simulink model "E55_1030"  (R2019b)
settings: Solver=FixedStepDiscrete  StartTime=0.0  StopTime=10  FixedStep=0.0005  RelTol=1e-3  EnableMultiTasking=on
InitFcn:
  | ecucoder_canfd
  | load('DATA_Plimit.mat')
  | a=0.775;
  | b=0.775;
  | kf=-50000;
  | kr=-50000;
  | m=226+75;
  | Iz=100;
  | u=0.85;
  | g=9.8;
  | L=a+b;
  | xi=0.1;
  | r=0.226;
  | Lw=1.171;
  | Tm=21;
  | i=15.9;
  | Jw=0.504;
  | Pmax=20000;
  | mw=19.3;
  | mb=148.9+75;
  | hg=0.280;
model workspace (MAT data in the model file):
  Initial_Steer_Position = 0
values from neighbouring files (symbols this model uses):
  SOC = [2.5 5 7.5 10 20 30 40 50 60 70 80 90 ... (14 elements, 14x1)]    [DATA_Plimit.mat]
  SOC_Discharge = [2.04592350211 2.57821618825 3.10671863859 3.63118835861 4.15200192786 4.66837694959 5.18149950051 5.69046162564 6.19532286188 6.696400261 7.19347596839 7.68712157998 ... (473 elements, 1x473)]    [DATA_Plimit.mat]
  VOLTAGE = [459.1488 476.0844 485.9448 487.344 492.822 498.8016 503.382 509.1108 518.8128 531.2472 544.5132 558.4656 ... (14 elements, 14x1)]    [DATA_Plimit.mat]
undefined symbols (not defined in the file or in its folder): DiscIntNeverNeededParam, H, HALL10, HALL6, HALL7, HALL8, HALL9, HPWM1, HPWM3, I_AN05_5V, I_AN07_5V, I_AN08_5V, I_AN09_5V, I_AN10_5V, I_SW11_H, I_SW12_H, I_SW13_H, I_SW14_H, I_SW15_H, I_SW16_H, I_SW17_H, I_SW18_H, I_SW19_H, LS1A2, O_HS1A2, O_HS1A8
libraries: ec311lib x152, simulink x92, canmsglib x30, canfdmsglib x2
(part 1 of 6)
settings Model: PacingRate=0.100000  Creator=Bobbby  LastModifiedBy=Administrator
settings OptimizationCC: DefaultParameterBehavior=Inlined  InlineInvariantSignals=on  EnhancedBackFolding=on  ExpressionFolding=off  PassReuseOutputArgsAs=Individual arguments  RollThreshold=65  StateBitsets=on  DataBitsets=on  ZeroExternalMemoryAtStartup=off  ZeroInternalMemoryAtStartup=off  EfficientFloat2IntCast=on  OptimizeBlockOrder=speed  DifferentSizesBufferReuse=on  EfficientTunableParamExpr=on
settings DebuggingCC: InheritedTsInSrcMsg=none  ParameterTunabilityLossMsg=error  UnconnectedInputMsg=none  UnconnectedOutputMsg=none  UnconnectedLineMsg=none  SFMachineParentedDataDiag=error
settings HardwareCC: ProdBitPerPointer=32  ProdBitPerSizeT=32  ProdBitPerPtrDiffT=32  ProdLargestAtomicInteger=Long  ProdLargestAtomicFloat=Double  ProdWordSize=32  ProdHWDeviceType=ARM Compatible->ARM Cortex
settings SFSimCC: MATLABDynamicMemAlloc=off  CustomCodeUndefinedFunction=UseInterfaceOnly
settings RTWCC: Description=Target for EC311  SystemTargetFile=ec311.tlc  MakeCommand=make_rtw optimized_fixed_point=1  GenerateMakefile=off  TemplateMakefile=ec311_lcc.tmf  PostCodeGenCommand=ec311_pst_s2(buildInfo)  GenerateReport=on  IncludeHyperlinkInReport=on  LaunchReport=on
settings CodeAppCC: ForceParamTrailComments=on  IgnoreCustomStorageClasses=off  OperatorAnnotations=on  SimulinkDataObjDesc=on  SFDataObjDesc=on  InsertBlockDesc=on
settings STFCustomTargetCC: TargetLangStandard=C99 (ISO)  MultiwordLength=256  IncludeMdlTerminateFcn=off  CombineOutputUpdateFcns=on  SuppressErrorStatus=on  ERTCustomFileBanners=on  SupportNonFinite=off  SupportContinuousTime=off  SupportNonInlinedSFcns=off  RemoveResetFunc=on  MATLABClassNameForMDSCustomization=Simulink.SoftwareTarget.ERTCustomization  SystemTargetFile=ec311.tlc
settings ERTTargetCC: TargetLangStandard=C99 (ISO)  ParMdlRefBuildCompliant=off  CompOptLevelCompliant=off  ConcurrentExecutionCompliant=off  IncludeMdlTerminateFcn=off  SuppressErrorStatus=on  SupportNonFinite=off  ModelStepFunctionPrototypeControlCompliant=off  CPPClassGenCompliant=off  UseToolchainInfoCompliant=off  GenerateASAP2=on  InlinedParameterPlacement=NonHierarchical  ERTSrcFileBannerTemplate=ec311_code_template.cgt  ERTHdrFileBannerTemplate=ec311_code_template.cgt  ERTDataSrcFileTemplate=ec311_code_template.cgt  ERTDataHdrFileTemplate=ec311_code_template.cgt  ERTCustomFileTemplate=ec311_file_process.tlc

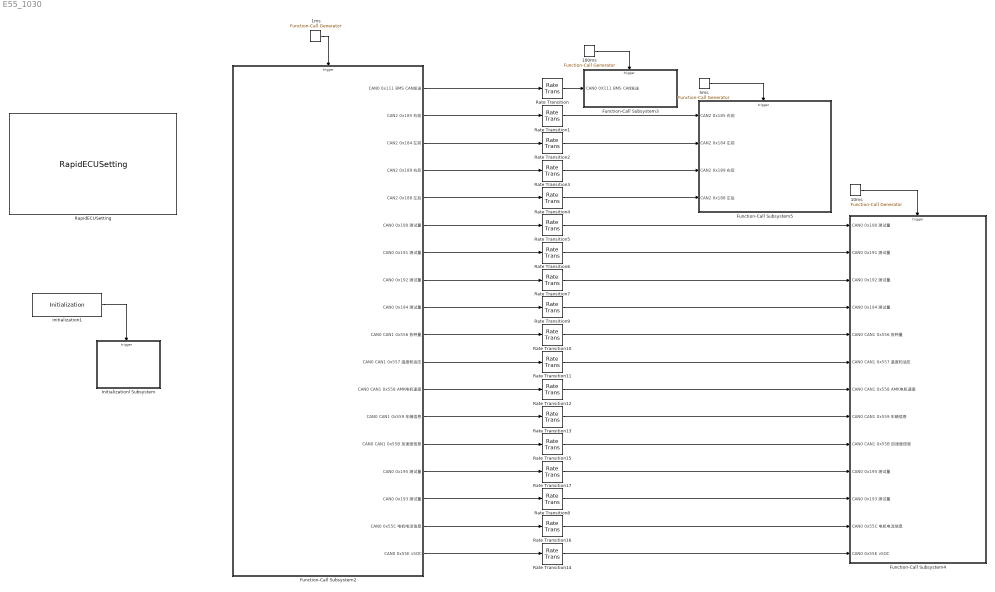
== system E55_1030 ==
  100ms : simulink/Ports & Subsystems/Function-Call Generator  sample_time=0.1  numberOfIterations=1
  10ms : simulink/Ports & Subsystems/Function-Call Generator  sample_time=0.01  numberOfIterations=1
  1ms : simulink/Ports & Subsystems/Function-Call Generator  sample_time=0.001  numberOfIterations=1
  5ms : simulink/Ports & Subsystems/Function-Call Generator  sample_time=0.005  numberOfIterations=1
  Function-Call Subsystem2 : Subsystem  TreatAsAtomicUnit=on
  Function-Call Subsystem3 : Subsystem  TreatAsAtomicUnit=on
  Function-Call Subsystem4 : Subsystem  TreatAsAtomicUnit=on
  Function-Call Subsystem5 : Subsystem  TreatAsAtomicUnit=on
  Initialization1 : ec311lib/RapidECU_U34/08MCUManagement/Initialization
      settings: SourceProductName=ECUCoder for S32K311
  Initializationl Subsystem : Subsystem  TreatAsAtomicUnit=on
  RapidECUSetting : ec311lib/RapidECU_U34/RapidECUSetting
      link override CAN: fmode=1  fpl=64  emode=1  epl=64  bmode=0  bpl=8
      settings: SourceProductName=ECUCoder for S32K311
  Rate Transition{,1..17} (18 alike) : RateTransition
  wires:
  Initialization1/1 -> Initializationl Subsystem/Trigger
  100ms/1 -> Function-Call Subsystem3/Trigger
  Function-Call Subsystem2/1(CAN0 0x111 BMS CAN发送) -> Rate Transition/1
  10ms/1 -> Function-Call Subsystem4/Trigger
  Function-Call Subsystem2/2(CAN2 0x185 右前) -> Rate Transition1/1
  Function-Call Subsystem2/3(CAN2 0x184 左前) -> Rate Transition2/1
  Function-Call Subsystem2/4(CAN2 0x189 右后) -> Rate Transition3/1
  Function-Call Subsystem2/5(CAN2 0x188 左后) -> Rate Transition4/1
  Rate Transition1/1 -> Function-Call Subsystem5/1(CAN2 0x185 右前)
  Rate Transition2/1 -> Function-Call Subsystem5/2(CAN2 0x184 左前)
  Rate Transition3/1 -> Function-Call Subsystem5/3(CAN2 0x189 右后)
  Rate Transition4/1 -> Function-Call Subsystem5/4(CAN2 0x188 左后)
  Function-Call Subsystem2/6(CAN0 0x190 测试量) -> Rate Transition5/1
  Function-Call Subsystem2/7(CAN0 0x191 测试量) -> Rate Transition6/1
  Function-Call Subsystem2/8(CAN0 0x192 测试量) -> Rate Transition7/1
  Function-Call Subsystem2/9(CAN0 0x194 测试量) -> Rate Transition9/1
  Rate Transition5/1 -> Function-Call Subsystem4/1(CAN0 0x190 测试量)
  Rate Transition6/1 -> Function-Call Subsystem4/2(CAN0 0x191 测试量)
  Rate Transition7/1 -> Function-Call Subsystem4/3(CAN0 0x192 测试量)
  Rate Transition9/1 -> Function-Call Subsystem4/4(CAN0 0x194 测试量)
  Function-Call Subsystem2/10(CAN0 CAN1 0x556 各种量) -> Rate Transition10/1
  Function-Call Subsystem2/11(CAN0 CAN1 0x557 温度和油压) -> Rate Transition11/1
  Function-Call Subsystem2/12(CAN0 CAN1 0x558 AMK电机速度) -> Rate Transition12/1
  Function-Call Subsystem2/13(CAN0 CAN1 0x559 车辆信息) -> Rate Transition13/1
  Function-Call Subsystem2/14(CAN0 CAN1 0x55B 加速度信息) -> Rate Transition15/1
  Rate Transition10/1 -> Function-Call Subsystem4/5(CAN0 CAN1 0x556 各种量)
  Rate Transition11/1 -> Function-Call Subsystem4/6(CAN0 CAN1 0x557 温度和油压)
  Rate Transition12/1 -> Function-Call Subsystem4/7(CAN0 CAN1 0x558 AMK电机速度)
  Rate Transition13/1 -> Function-Call Subsystem4/8(CAN0 CAN1 0x559 车辆信息)
  Rate Transition15/1 -> Function-Call Subsystem4/9(CAN0 CAN1 0x55B 加速度信息)
  5ms/1 -> Function-Call Subsystem5/Trigger
  Function-Call Subsystem2/15(CAN0 0x195 测试量) -> Rate Transition17/1
  Rate Transition17/1 -> Function-Call Subsystem4/10(CAN0 0x195 测试量)
  1ms/1 -> Function-Call Subsystem2/Trigger
  Function-Call Subsystem2/16(CAN0 0x193 测试量) -> Rate Transition8/1
  Rate Transition8/1 -> Function-Call Subsystem4/11(CAN0 0x193 测试量)
  Function-Call Subsystem2/17(CAN0 0x55C 电机电流信息) -> Rate Transition16/1
  Rate Transition16/1 -> Function-Call Subsystem4/12(CAN0 0x55C 电机电流信息)
  Rate Transition/1 -> Function-Call Subsystem3/1(CAN0 0X111 BMS CAN发送)
  Function-Call Subsystem2/18(CAN0 0x55E vSOC) -> Rate Transition14/1
  Rate Transition14/1 -> Function-Call Subsystem4/13(CAN0 0x55E vSOC)
